simulink model "super_regen_1"  (Simulink 7.4)
settings: Solver=ode45  StartTime=0.0  StopTime=8/1000  MaxStep=1/(5*Fcarrier)  RelTol=1e-3
PreLoadFcn:
  | Fcarrier=10e6;
  | C = 50e-12;
  | R = 1000;
  | Fmod=1000;
  | Fquench = 10e3;
libraries: powerlib x7, simulink x3
settings Model: Creator=Owner  LastModifiedBy=Dick
settings OptimizationCC: InitFltsAndDblsToZero=on

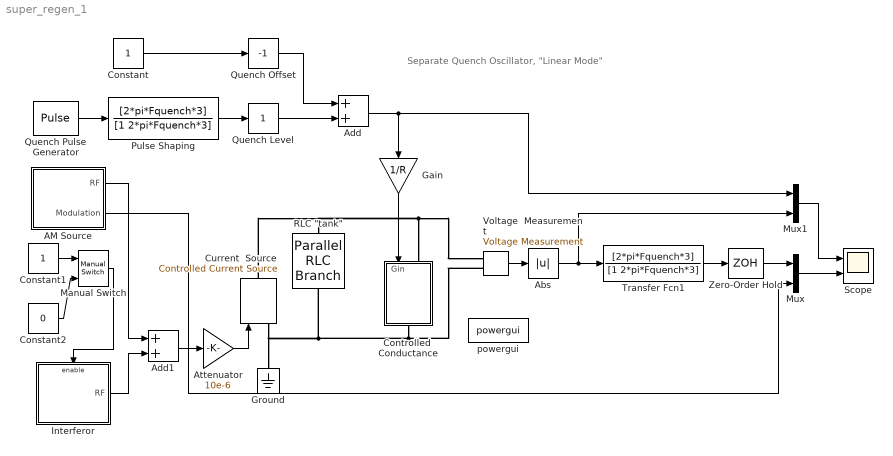
== system super_regen_1 ==
  note: Separate Quench Oscillator, "Linear Mode"
  AM Source : Subsystem
  Abs : Abs  OutDataType=sfix(16)  OutScaling=2^0
  Add : Sum  OutDataType=sfix(16)  OutScaling=2^-10
  Add1 : Sum  OutDataType=sfix(16)  OutScaling=2^-10
  Attenuator : Gain  Gain=10e-6  ParameterDataType=sfix(16)  ParameterScaling=2^0  OutDataType=sfix(16)  OutScaling=2^0
  Constant : Constant  OutDataType=sfix(16)  OutScaling=2^0
  Constant1 : Constant  OutDataType=sfix(16)  OutScaling=2^0
  Constant2 : Constant  Value=0  OutDataType=sfix(16)  OutScaling=2^0
  Controlled  Conductance : Subsystem
  Current  Source : powerlib/Electrical Sources/Controlled Current Source  DialogController=POWERSYS.PowerSysDialog  SystemSampleTime=-1  Initialize=on  Source_Type=DC  Amplitude=0  Phase=0  Frequency=0  Measurements=None
  Gain : Gain  Gain=1/R  ParameterDataType=sfix(16)  ParameterScaling=2^0  OutDataType=sfix(16)  OutScaling=2^0
  Ground : powerlib/Elements/Ground  DialogController=POWERSYS.PowerSysDialog  PhysicalDomain=powersysdomain  SubClassName=unknown  LeftPortType=p1  RightPortType=p1  LConnTagsString=a
  Interferor : Subsystem
  Manual Switch : simulink/Signal Routing/Manual Switch  SystemSampleTime=-1  sw=0  action=0  varsize=off
  Mux : Mux  Inputs=2
  Mux1 : Mux  Inputs=2
  Pulse Shaping : TransferFcn  Numerator=[2*pi*Fquench*3]  Denominator=[1 2*pi*Fquench*3]
  Quench Level : simulink/Math Operations/Slider Gain  SystemSampleTime=-1  low=0  gain=1  high=2
  Quench Offset : simulink/Math Operations/Slider Gain  SystemSampleTime=-1  low=-1.1  gain=-1  high=-0.8
  Quench Pulse Generator : DiscretePulseGenerator  PulseType=Time based  Amplitude=1  Period=1/Fquench  PulseWidth=50  PhaseDelay=0/Fquench  SampleTime=1
  "RLC \"tank\"" : powerlib/Elements/Parallel RLC Branch  DialogController=POWERSYS.PowerSysDialog  PhysicalDomain=powersysdomain  SubClassName=unknown  LeftPortType=p1  RightPortType=p1  LConnTagsString=a  RConnTagsString=__new0  BranchType=RLC  Resistance=R  Inductance=1/(((2*pi*Fcarrier)^2) *C)  SetiL0=off  InitialCurrent=0  Capacitance=C  Setx0=off  InitialVoltage=0  Measurements=None
  Scope : Scope  NumInputPorts=2
      settings: TimeRange=0.008  YMin=-1~-1  YMax=6~3  MaxDataPoints=1e6
  Transfer Fcn1 : TransferFcn  Numerator=[2*pi*Fquench*3]  Denominator=[1 2*pi*Fquench*3]
  Voltage  Measurement : powerlib/Measurements/Voltage Measurement  DialogController=POWERSYS.PowerSysDialog  SystemSampleTime=-1  PhasorSimulation=off  OutputType=Complex  PSBequivalent=0
  Zero-Order Hold : ZeroOrderHold  SampleTime=1/Fquench
  powergui : powerlib/powergui  SystemSampleTime=-1  SimulationMode=Continuous  SampleTime=50e-6  frequency=60  SPID=off  DisableSnubberDevices=off  DisableRonSwitches=off  DisableVfSwitches=off  SwTol=0  Interpol=off  frequencyindice=0  echomessages=off  HookPort=off  DisplayEquations=off  FunctionMessages=off  EnableUseOfTLC=off  x0status=blocks  RestoreLinks=warning  Frange=[0:2:500]  Ylog=off  Xlog=on  ShowGrid=off  save=off  variable=ZData  ZoomFFT=on  StartTime=0.0  cycles=1  DisplayStyle=1  fundamental=60  FreqAxis=off  MaxFrequency=1000  frequencyindicesteady=1  RmsSteady=1  display=off  Ts=0  methode=off
  wires:
  Pulse Shaping/1 -> Quench Level/1
  Quench Pulse Generator/1 -> Pulse Shaping/1
  Quench Level/1 -> Add/2
  Constant/1 -> Quench Offset/1
  Quench Offset/1 -> Add/1
  Add/1 -> Gain/1, Mux1/1
  Gain/1 -> Controlled  Conductance/1(Gin)
  Attenuator/1 -> Current  Source/1
  Abs/1 -> Transfer Fcn1/1, Mux1/2
  Transfer Fcn1/1 -> Zero-Order Hold/1
  Voltage  Measurement/1 -> Abs/1
  Mux/1 -> Scope/2
  Mux1/1 -> Scope/1
  Zero-Order Hold/1 -> Mux/1
  AM Source/2(Modulation) -> Mux/2
  Add1/1 -> Attenuator/1
  Interferor/1(RF) -> Add1/2
  AM Source/1(RF) -> Add1/1
  Constant1/1 -> Manual Switch/1
  Constant2/1 -> Manual Switch/2
  Manual Switch/1 -> Interferor/Enable
  connections:
  Current  Source/RConn1 -- "RLC \"tank\""/LConn1 -- Voltage  Measurement/LConn1 -- Controlled  Conductance/LConn1
  Voltage  Measurement/LConn2 -- "RLC \"tank\""/RConn1 -- Current  Source/LConn1 -- Ground/LConn1 -- Controlled  Conductance/RConn1

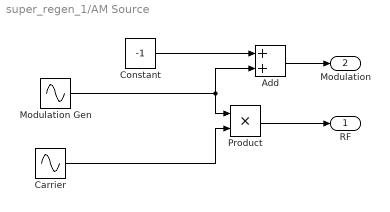
== system super_regen_1/AM Source ==
  Add : Sum  OutDataType=sfix(16)  OutScaling=2^-10
  Carrier : Sin  Amplitude=1  Bias=0  Frequency=Fcarrier*2*pi  Phase=0  Samples=10  SampleTime=0  Offset=0
  Constant : Constant  Value=-1  OutDataType=sfix(16)  OutScaling=2^0
  Modulation Gen : Sin  Amplitude=1  Bias=1  Frequency=Fmod*2*pi  Phase=0  Samples=10  SampleTime=0  Offset=0
  Product : Product  OutDataType=sfix(16)  OutScaling=2^0  RndMeth=Zero
  RF : Outport
  Modulation : Outport  Port=2
  wires:
  Modulation Gen/1 -> Product/1, Add/2
  Carrier/1 -> Product/2
  Product/1 -> RF/1
  Add/1 -> Modulation/1
  Constant/1 -> Add/1

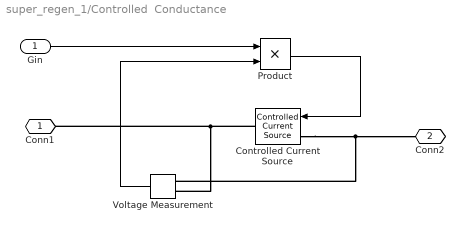
== system super_regen_1/Controlled  Conductance ==
  Gin : Inport  OutDataType=sfix(16)  OutScaling=2^0
  Controlled Current Source : powerlib/Electrical Sources/Controlled Current Source  DialogController=POWERSYS.PowerSysDialog  SystemSampleTime=-1  Initialize=on  Source_Type=AC  Amplitude=0  Phase=0  Frequency=0  Measurements=None
  Product : Product  OutDataType=sfix(16)  OutScaling=2^0  RndMeth=Zero
  Voltage Measurement : powerlib/Measurements/Voltage Measurement  DialogController=POWERSYS.PowerSysDialog  SystemSampleTime=-1  PhasorSimulation=off  OutputType=Complex  PSBequivalent=0
  Conn1 : PMIOPort  Port=1  Side=Left
  Conn2 : PMIOPort  Port=2  Side=Right
  wires:
  Gin/1 -> Product/1
  Product/1 -> Controlled Current Source/1
  Voltage Measurement/1 -> Product/2
  connections:
  Controlled Current Source/LConn1 -- Conn2/RConn1 -- Voltage Measurement/LConn1
  Controlled Current Source/RConn1 -- Conn1/RConn1 -- Voltage Measurement/LConn2

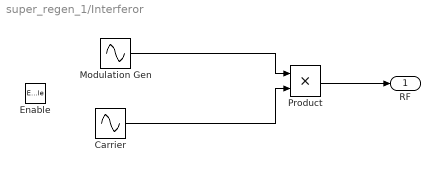
== system super_regen_1/Interferor ==
  Enable : EnablePort
  Carrier : Sin  Amplitude=1  Bias=0  Frequency=(Fcarrier+200e3)*2*pi  Phase=0  Samples=10  SampleTime=0  Offset=0
  Modulation Gen : Sin  Amplitude=1  Bias=1  Frequency=Fmod*2*pi*2  Phase=0  Samples=10  SampleTime=0  Offset=0
  Product : Product  OutDataType=sfix(16)  OutScaling=2^0  RndMeth=Zero
  RF : Outport
  wires:
  Product/1 -> RF/1
  Carrier/1 -> Product/2
  Modulation Gen/1 -> Product/1
